simulink model "EV_fault_management"  (R2025b)
settings: Solver=VariableStepAuto  StartTime=0.0  StopTime=10.0  RelTol=1e-3
settings Model: Creator=Puki  LastModifiedBy=Puki

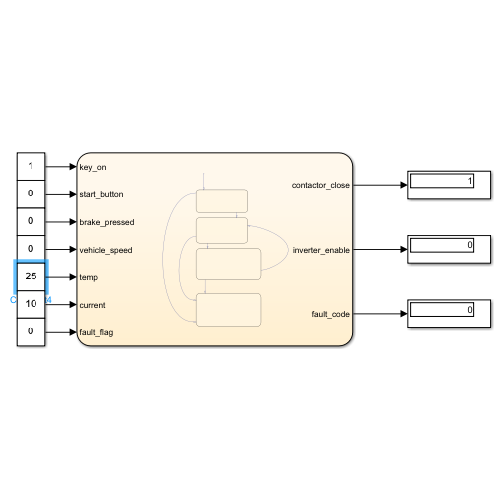
[thumbnail: Simulink's stored preview of the top-level diagram]
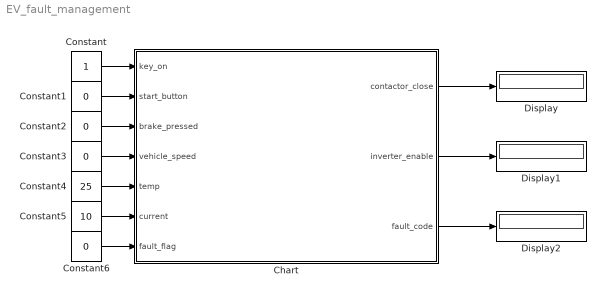
== system EV_fault_management ==
  Chart : Stateflow chart  TreatAsAtomicUnit=on
  Constant : Constant
  Constant{1..3,6} (4 alike) : Constant  Value=0
  Constant4 : Constant  Value=25
  Constant5 : Constant  Value=10
  Display : Display
  Display1 : Display
  Display2 : Display
  wires:
  Constant/1 -> Chart/1(key_on)
  Constant1/1 -> Chart/2(start_button)
  Constant2/1 -> Chart/3(brake_pressed)
  Constant3/1 -> Chart/4(vehicle_speed)
  Constant4/1 -> Chart/5(temp)
  Constant5/1 -> Chart/6(current)
  Constant6/1 -> Chart/7(fault_flag)
  Chart/1(contactor_close) -> Display/1
  Chart/3(fault_code) -> Display2/1
  Chart/2(inverter_enable) -> Display1/1

== stateflow chart EV_fault_management/Chart ==
  state Off
    entry:
    contactor_close = 0;
    inverter_enable = 0;
    fault_code = 0;
  state Standby
    entry:
    contactor_close = 1;
    inverter_enable = 0;
    fault_code = 0;
  state Drive
    entry:
    contactor_close = 1;
    inverter_enable = 1;
    fault_code = 0;
  state Fault
    entry:
    contactor_close = 0;
    inverter_enable = 0;
    fault_code = 1;
  (default) -> Off
  Off -> Fault [order 1] : [fault_flag == 1 || temp > 80 || current > 250]
  Off -> Standby [order 2] : [key_on ==1 && fault_flag == 0]
  Drive -> Standby [order 2] : [vehicle_speed == 0 && brake_pressed == 1]
  Standby -> Fault [order 1] : [fault_flag == 1 || temp > 80 || current > 250]
  Standby -> Drive [order 2] : [brake_pressed == 1 && start_button == 1]
  Drive -> Fault [order 1] : [fault_flag == 1 || temp > 80 || current > 250]
  data: key_on input; start_button input; brake_pressed input; vehicle_speed input; temp input; current input; fault_flag input; contactor_close output; inverter_enable output; fault_code output
